simulink model "puma_dy_create_model_ext"  (R2015b)
settings: Solver=FixedStepAuto  StartTime=0.0  StopTime=5  FixedStep=0.01  RelTol=1e-3
values from neighbouring files (symbols this model uses):
  g = 9.80665    [puma_gen_traj_and_mass_param_ext.m]
  ic1 = [ 77887.93599651e-6, -0.00013107e-6, 0.00000935e-6 ... (first row only)    [puma_gen_traj_and_mass_param_ext.m]
  ic2 = [ 214693.97411152e-6, 0, -9732.69714079e-6 ... (first row only)    [puma_gen_traj_and_mass_param_ext.m]
  ic3 = [ 155440.16360976e-6, -7644.06665755e-6, 0.00000000 ... (first row only)    [puma_gen_traj_and_mass_param_ext.m]
  ic4 = [ 2247.32396481e-6, 0.00000000, 0.00000000 ... (first row only)    [puma_gen_traj_and_mass_param_ext.m]
  ic5 = [103.66681738e-6, 0.00000001e-6, -0.00000014e-6 ... (first row only)    [puma_gen_traj_and_mass_param_ext.m]
  ic6 = [311.60326416e-6, -0.00000017e-6, 0.00000000 ... (first row only)    [puma_gen_traj_and_mass_param_ext.m]
  m1 = 12.65615427    [puma_gen_traj_and_mass_param_ext.m]
  m2 = 41.52453758    [puma_gen_traj_and_mass_param_ext.m]
  m3 = 9.95151214    [puma_gen_traj_and_mass_param_ext.m]
  m4 = 1.32832452    [puma_gen_traj_and_mass_param_ext.m]
  m5 = 0.21689844    [puma_gen_traj_and_mass_param_ext.m]
  m6 = 0.32891048    [puma_gen_traj_and_mass_param_ext.m]
  P112 = [ 0 d3 0 ]'    [puma_gen_traj_and_mass_param_ext.m]
  P223 = [ a2 0 0 ]'    [puma_gen_traj_and_mass_param_ext.m]
  P334 = [ a3 d4 0 ]'    [puma_gen_traj_and_mass_param_ext.m]
  P445 = [ 0 0 0 ]'    [puma_gen_traj_and_mass_param_ext.m]
  P556 = [ 0 0 0 ]'    [puma_gen_traj_and_mass_param_ext.m]
  P667 = [ 0 0 0 ]'    [puma_gen_traj_and_mass_param_ext.m]
  Pc111 = [ 0 18.97808196e-3 -4.26387031e-3 ]'    [puma_gen_traj_and_mass_param_ext.m]
  Pc222 = [ 70.91581478e-3 0.00000000 211.69489465e-3-d3 ]'    [puma_gen_traj_and_mass_param_ext.m]
  Pc333 = [ 17.56050216e-3 119.38037782e-3 0 ]'    [puma_gen_traj_and_mass_param_ext.m]
  Pc444 = [ 0 0 -32.52388888e-3 ]'    [puma_gen_traj_and_mass_param_ext.m]
  Pc555 = [ 0 -6.06453643e-3 0 ]'    [puma_gen_traj_and_mass_param_ext.m]
  Pc666 = [ 0 0 93.94499327e-3 ]'    [puma_gen_traj_and_mass_param_ext.m]
libraries: mblibv1 x29
settings Model: Creator=user  LastModifiedBy=qing.hao
settings SimMechanicsCC: VisOnUpdateDiagram=on  VisDuringSimulation=on  LastVizWinPosition=[1 41 1920 938]  CamPosition=[6.48278;4.07346;8.12681;]  CamTarget=[-0.751108;-0.0621973;-0.55549;]  CamUpVector=[-0.477891;-0.569017;0.669208;]  CamHeight=1.40512  VisBackgroundColor=[0.9;0.9;0.95;]  DefaultBodyColor=[1;0;0;]

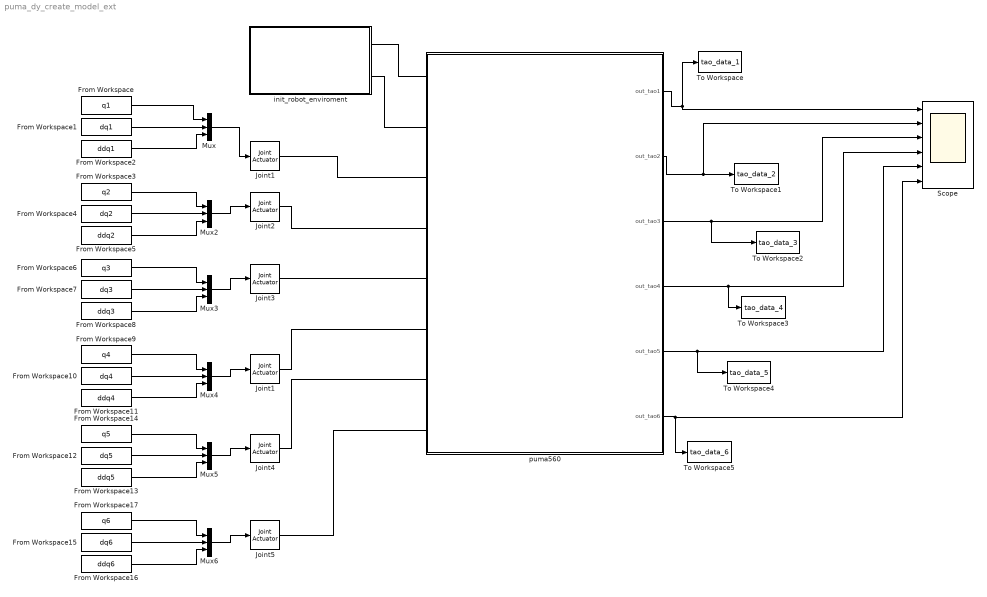
== system puma_dy_create_model_ext ==
  From Workspace : FromWorkspace  VariableName=q1  SampleTime=0.01
  From Workspace1 : FromWorkspace  VariableName=dq1  SampleTime=0.01
  From Workspace10 : FromWorkspace  VariableName=dq4  SampleTime=0.01
  From Workspace11 : FromWorkspace  VariableName=ddq4  SampleTime=0.01
  From Workspace12 : FromWorkspace  VariableName=dq5  SampleTime=0.01
  From Workspace13 : FromWorkspace  VariableName=ddq5  SampleTime=0.01
  From Workspace14 : FromWorkspace  VariableName=q5  SampleTime=0.01
  From Workspace15 : FromWorkspace  VariableName=dq6  SampleTime=0.01
  From Workspace16 : FromWorkspace  VariableName=ddq6  SampleTime=0.01
  From Workspace17 : FromWorkspace  VariableName=q6  SampleTime=0.01
  From Workspace2 : FromWorkspace  VariableName=ddq1  SampleTime=0.01
  From Workspace3 : FromWorkspace  VariableName=q2  SampleTime=0.01
  From Workspace4 : FromWorkspace  VariableName=dq2  SampleTime=0.01
  From Workspace5 : FromWorkspace  VariableName=ddq2  SampleTime=0.01
  From Workspace6 : FromWorkspace  VariableName=q3  SampleTime=0.01
  From Workspace7 : FromWorkspace  VariableName=dq3  SampleTime=0.01
  From Workspace8 : FromWorkspace  VariableName=ddq3  SampleTime=0.01
  From Workspace9 : FromWorkspace  VariableName=q4  SampleTime=0.01
  Joint{1..5} (5 alike) : mblibv1/Sensors &  Actuators/Joint Actuator  UpdateFromCAD=off  PhysicalDomain=Mechanical  PortType=blob  ActuationStyle=Motion  AngleUnits=deg  ArcVelocityUnits=deg/s  ArcAccelerationUnits=deg/s^2  CoordPositionUnits=m  VelocityUnits=m/s  AccelerationUnits=m/s^2  ForceUnits=N  TorqueUnits=N*m  ActiveIO=on  Width=3  DialogClass=MechanicalActuatorBlock  Primitive=R1  ReferenceFrame=Absolute (World)
  "Joint1 " : mblibv1/Sensors &  Actuators/Joint Actuator  UpdateFromCAD=off  PhysicalDomain=Mechanical  PortType=blob  ActuationStyle=Motion  AngleUnits=deg  ArcVelocityUnits=deg/s  ArcAccelerationUnits=deg/s^2  CoordPositionUnits=m  VelocityUnits=m/s  AccelerationUnits=m/s^2  ForceUnits=N  TorqueUnits=N*m  ActiveIO=on  Width=3  DialogClass=MechanicalActuatorBlock  Primitive=R1  ReferenceFrame=Absolute (World)
  Mux{,2..6} (6 alike) : Mux  Inputs=3
  Scope : Scope  NumInputPorts=6
  To Workspace : ToWorkspace  VariableName=tao_data_1  SaveFormat=Timeseries  SampleTime=-1
  To Workspace1 : ToWorkspace  VariableName=tao_data_2  SaveFormat=Timeseries  SampleTime=-1
  To Workspace2 : ToWorkspace  VariableName=tao_data_3  SaveFormat=Timeseries  SampleTime=-1
  To Workspace3 : ToWorkspace  VariableName=tao_data_4  SaveFormat=Timeseries  SampleTime=-1
  To Workspace4 : ToWorkspace  VariableName=tao_data_5  SaveFormat=Timeseries  SampleTime=-1
  To Workspace5 : ToWorkspace  VariableName=tao_data_6  SaveFormat=Timeseries  SampleTime=-1
  "init_robot_enviroment " : Subsystem
  puma560 : Subsystem
  wires:
  From Workspace/1 -> Mux/1
  From Workspace1/1 -> Mux/2
  From Workspace2/1 -> Mux/3
  Mux/1 -> "Joint1 "/1
  From Workspace3/1 -> Mux2/1
  From Workspace4/1 -> Mux2/2
  From Workspace5/1 -> Mux2/3
  Mux2/1 -> Joint2/1
  From Workspace6/1 -> Mux3/1
  From Workspace7/1 -> Mux3/2
  From Workspace8/1 -> Mux3/3
  Mux3/1 -> Joint3/1
  From Workspace9/1 -> Mux4/1
  From Workspace10/1 -> Mux4/2
  From Workspace11/1 -> Mux4/3
  Mux4/1 -> Joint1/1
  From Workspace14/1 -> Mux5/1
  From Workspace12/1 -> Mux5/2
  From Workspace13/1 -> Mux5/3
  Mux5/1 -> Joint4/1
  From Workspace17/1 -> Mux6/1
  From Workspace15/1 -> Mux6/2
  From Workspace16/1 -> Mux6/3
  Mux6/1 -> Joint5/1
  puma560/1(out_tao1) -> To Workspace/1, Scope/1
  puma560/2(out_tao2) -> To Workspace1/1, Scope/2
  puma560/3(out_tao3) -> To Workspace2/1, Scope/3
  puma560/4(out_tao4) -> To Workspace3/1, Scope/4
  puma560/5(out_tao5) -> To Workspace4/1, Scope/5
  puma560/6(out_tao6) -> To Workspace5/1, Scope/6
  connections:
  "Joint1 "/RConn1 -- puma560/LConn3
  puma560/LConn4 -- Joint2/RConn1
  puma560/LConn5 -- Joint3/RConn1
  Joint1/RConn1 -- puma560/LConn6
  Joint4/RConn1 -- puma560/LConn7
  puma560/LConn8 -- Joint5/RConn1
  puma560/LConn1 -- "init_robot_enviroment "/RConn1
  puma560/LConn2 -- "init_robot_enviroment "/RConn2

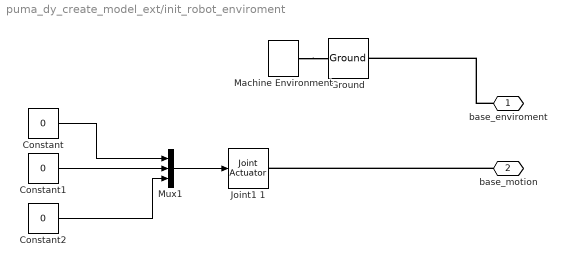
== system puma_dy_create_model_ext/init_robot_enviroment  ==
  Constant : Constant  Value=0
  Constant1 : Constant  Value=0
  Constant2 : Constant  Value=0
  Ground : mblibv1/Bodies/Ground  UpdateFromCAD=off  LeftPortType=env  RightPortType=workingframe  PhysicalDomain=Mechanical  DialogClass=GroundBlock  CoordPosition=[0 0 0]  CoordPositionUnits=m  StateVectorMgrId=3  MachineId=[4 0]  ShowEnvPort=on  ParameterChecksum=[2230059467, 3484987599, 1936103791, 2977691241]  TopologyChecksum=[2683286288, 4268472829, 915100555, 2393938141]
  Joint1 1 : mblibv1/Sensors &  Actuators/Joint Actuator  UpdateFromCAD=off  PhysicalDomain=Mechanical  PortType=blob  ActuationStyle=Motion  AngleUnits=deg  ArcVelocityUnits=deg/s  ArcAccelerationUnits=deg/s^2  CoordPositionUnits=m  VelocityUnits=m/s  AccelerationUnits=m/s^2  ForceUnits=N  TorqueUnits=N*m  ActiveIO=on  Width=3  DialogClass=MechanicalActuatorBlock  Primitive=R1  ReferenceFrame=Absolute (World)
  Machine Environment : mblibv1/Bodies/Machine Environment  PortType=env  PhysicalDomain=Mechanical  DialogTemplateClass=MECH.MachineEnvironment  SyncWhenCopied=off  Gravity=[0 0 -g]  GravityUnits=m/s^2  GravityAsSignal=off  Dimensionality=Auto-detect  AnalysisType=Forward dynamics  LinearAssemblyTolerance=1e-3  LinearAssemblyToleranceUnits=mm  AngularAssemblyTolerance=1e-3  AngularAssemblyToleranceUnits=deg  ConstraintSolverType=Stabilizing  ConstraintRelTolerance=1e-4  ConstraintAbsTolerance=1e-4  UseRobustSingularityHandling=off  RedundancyAnalysisToleranceType=Automatically select tolerance  RedundancyAnalysisTolerance=1e-14  StatePerturbationType=Fixed  PerturbationSize=1e-5  VisualizeMachine=on  BodyVisualizationType=Use model default body geometries  BodyColorSelMode=Use model default  DefaultBodyColor=[1 0 0]
  Mux1 : Mux  Inputs=3
  base_enviroment : PMIOPort  Port=1  Side=Right
  base_motion : PMIOPort  Port=2  Side=Right
  wires:
  Constant1/1 -> Mux1/2
  Constant/1 -> Mux1/1
  Constant2/1 -> Mux1/3
  Mux1/1 -> Joint1 1/1
  connections:
  Machine Environment/RConn1 -- Ground/LConn1
  base_motion/RConn1 -- Joint1 1/RConn1
  base_enviroment/RConn1 -- Ground/RConn1

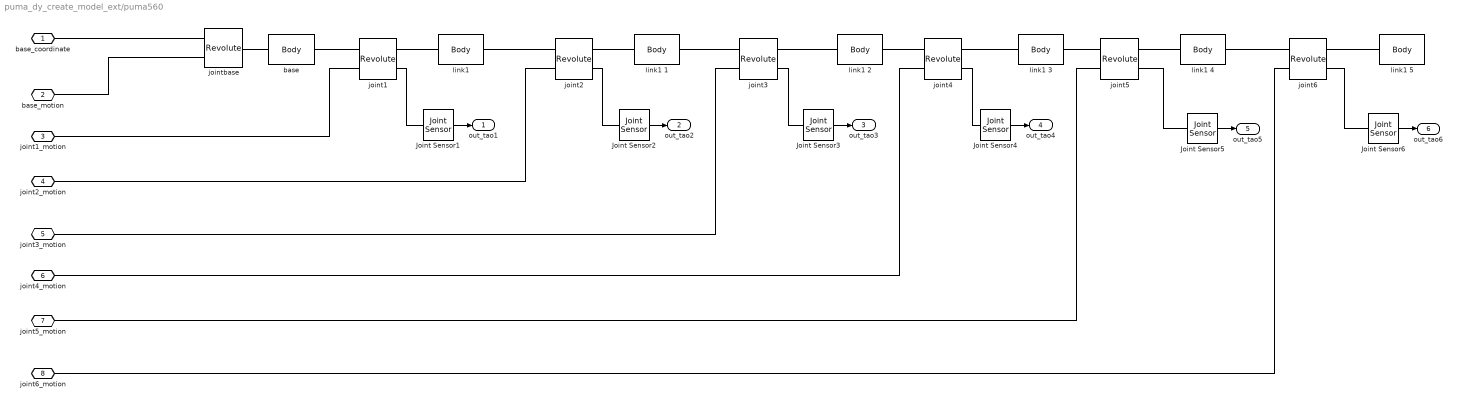
== system puma_dy_create_model_ext/puma560 ==
  Joint Sensor{1..6} (6 alike) : mblibv1/Sensors &  Actuators/Joint Sensor  UpdateFromCAD=off  PhysicalDomain=Mechanical  PortType=blob  Muxed=on  Pose=off  Angle=off  AngleUnits=deg  ArcVelocity=off  ArcVelocityUnits=deg/s  ArcAcceleration=off  ArcAccelerationUnits=deg/s^2  CoordPosition=on  CoordPositionUnits=m  Velocity=off  VelocityUnits=m/s  Acceleration=off  AccelerationUnits=m/s^2  Quaternion=on  QuaternionDT=off  QuaternionDDT=off  QuaternionUnits=off  OutputVector=[1]  ActiveIO=on  Width=1  DialogClass=MechanicalSensorBlock  Primitive=R1  Force=off  ForceUnits=N  Torque=on  TorqueUnits=N*m  ReferenceFrame=Absolute (World)  ReactionSensedSide=Base  ReactionReferenceFrame=Absolute (World)  ReactionForce=off  ReactionForceUnits=N  ReactionMoment=off  ReactionMomentUnits=N*m
  "base " : mblibv1/Bodies/Body  LConnTagsString=CS1  RConnTagsString=CS2  UpdateFromCAD=off  DialogClass=MechanicalBodyBlock  Mass=1  MassUnits=kg  InertiaUnits=kg*m^2  Inertia=eye(3)  Shape=Cylinder  ShapeDims=[1 1]  ShapeUnits=m  ShapeUse=false  Density=1  DensityUnits=kg/m^3  DensityUse=false  GraphicsMode=GFXFILE  GraphicsFileName=.\model\RobotPart0.STL  BodyColorSelMode=COLORPALETTE  BodyColor=[0.87059 0.4902 0]  AttachedToCS=CS3  CG=Left$CG$[0 0 300]$WORLD$WORLD$mm$[0 0 0]$Euler X-Y-Z$deg$WORLD$false$none  WorkingFrames="Left$CS1$[0 0 0]$World$World$mm$[0 0 0]$Euler X-Y-Z$deg$WORLD$true$none#Right$CS2$[0 0  633.57]$World$World$mm$[0 0 0]$Euler X-Y-Z$deg$WORLD$true$none#Right$CS3$[0 -234  0]$World$World$mm$[0 0 0]$Euler X-Y-Z$deg$WORLD$false$none"  CGPos=[0 0 300]  CGRot=[0 0 0]  CS0Pos=[]  CS0Rot=[]  CS1Pos=[0 0 0]  CS1Rot=[0 0 0]  CS2Pos="[0 0  633.57]"  CS2Rot=[0 0 0]  CS3Pos="[0 -234  0]"  CS3Rot=[0 0 0]  CS4Pos=[]  CS4Rot=[]  CS5Pos=[]  CS5Rot=[]  CS6Pos=[]  CS6Rot=[]  CS7Pos=[]  CS7Rot=[]  CS8Pos=[]  CS8Rot=[]  CS9Pos=[]  CS9Rot=[]  CS10Pos=[]  CS10Rot=[]  CS11Pos=[]  CS11Rot=[]  CS12Pos=[]  CS12Rot=[]  CS13Pos=[]  CS13Rot=[]  CS14Pos=[]  CS14Rot=[]  CS15Pos=[]  CS15Rot=[]  CS16Pos=[]  CS16Rot=[]  CS17Pos=[]  CS17Rot=[]  CS18Pos=[]  CS18Rot=[]  CS19Pos=[]  CS19Rot=[]  CS20Pos=[]  CS20Rot=[]
  joint{1..6} (6 alike) : mblibv1/Joints/Revolute  LConnTagsString=__newl0|SA1  RConnTagsString=__newr0|SA1  UpdateFromCAD=off  NumSAPorts=2  CutJoint=off  MarkAsCut=off  Primitives=prismatic  PrimitiveProps=R1$Base$[0 0 1]$revolute  DialogClass=JointBlock  R1Axis=[0 0 1]
  jointbase : mblibv1/Joints/Revolute  LConnTagsString=__newl0|SA1  RConnTagsString=__newr0  UpdateFromCAD=off  NumSAPorts=1  CutJoint=off  MarkAsCut=off  Primitives=prismatic  PrimitiveProps=R1$World$[0 0 1]$revolute  DialogClass=JointBlock  R1Axis=[0 0 1]
  "link1 " : mblibv1/Bodies/Body  LConnTagsString=CS1  RConnTagsString=CS2  UpdateFromCAD=off  DialogClass=MechanicalBodyBlock  Mass=m1  MassUnits=kg  InertiaUnits=kg*m^2  Inertia=ic1  Shape=Cylinder  ShapeDims=[1 1]  ShapeUnits=m  ShapeUse=false  Density=1  DensityUnits=kg/m^3  DensityUse=false  GraphicsMode=GFXFILE  GraphicsFileName=.\model\RobotPart1.STL  BodyColorSelMode=COLORPALETTE  BodyColor=[1 1 0]  AttachedToCS=CS3  CG=Left$CG$Pc111'*1000$CS1$CS1$mm$[0 0 0]$Euler X-Y-Z$deg$CS1$false$none  WorkingFrames=Left$CS1$[0 0 0]$Adjoining$Adjoining$mm$[0 0 0]$Euler X-Y-Z$deg$Adjoining$true$none#Right$CS2$P112'*1000$CS1$CS1$mm$[-90 0 0]$Euler X-Y-Z$deg$CS1$true$none#Right$CS3$[0 -568 0]$World$World$mm$[0 0 0]$Euler X-Y-Z$deg$World$false$none  CGPos=Pc111'*1000  CGRot=[0 0 0]  CS0Pos=[]  CS0Rot=[]  CS1Pos=[0 0 0]  CS1Rot=[0 0 0]  CS2Pos=P112'*1000  CS2Rot=[-90 0 0]  CS3Pos=[0 -568 0]  CS3Rot=[0 0 0]  CS4Pos=[]  CS4Rot=[]  CS5Pos=[]  CS5Rot=[]  CS6Pos=[]  CS6Rot=[]  CS7Pos=[]  CS7Rot=[]  CS8Pos=[]  CS8Rot=[]  CS9Pos=[]  CS9Rot=[]  CS10Pos=[]  CS10Rot=[]  CS11Pos=[]  CS11Rot=[]  CS12Pos=[]  CS12Rot=[]  CS13Pos=[]  CS13Rot=[]  CS14Pos=[]  CS14Rot=[]  CS15Pos=[]  CS15Rot=[]  CS16Pos=[]  CS16Rot=[]  CS17Pos=[]  CS17Rot=[]  CS18Pos=[]  CS18Rot=[]  CS19Pos=[]  CS19Rot=[]  CS20Pos=[]  CS20Rot=[]
  link1 1 : mblibv1/Bodies/Body  LConnTagsString=CS1  RConnTagsString=CS2  UpdateFromCAD=off  DialogClass=MechanicalBodyBlock  Mass=m2  MassUnits=kg  InertiaUnits=kg*m^2  Inertia=ic2  Shape=Cylinder  ShapeDims=[1 1]  ShapeUnits=m  ShapeUse=false  Density=1  DensityUnits=kg/m^3  DensityUse=false  GraphicsMode=GFXFILE  GraphicsFileName=.\model\RobotPart2.STL  BodyColorSelMode=COLORPALETTE  BodyColor=[0.23137 0.44314 0.33726]  AttachedToCS=CS3  CG=Left$CG$Pc222'*1000$CS1$CS1$mm$[0 0 0]$Euler X-Y-Z$deg$CS1$false$none  WorkingFrames=Left$CS1$[0 0 0]$Adjoining$Adjoining$mm$[0 0 0]$Euler X-Y-Z$deg$Adjoining$true$none#Right$CS2$P223'*1000$CS1$CS1$mm$[0 0 0]$Euler X-Y-Z$deg$CS1$true$none#Right$CS3$[0 -568 0]$World$World$mm$[0 0 0]$Euler X-Y-Z$deg$World$false$none  CGPos=Pc222'*1000  CGRot=[0 0 0]  CS0Pos=[]  CS0Rot=[]  CS1Pos=[0 0 0]  CS1Rot=[0 0 0]  CS2Pos=P223'*1000  CS2Rot=[0 0 0]  CS3Pos=[0 -568 0]  CS3Rot=[0 0 0]  CS4Pos=[]  CS4Rot=[]  CS5Pos=[]  CS5Rot=[]  CS6Pos=[]  CS6Rot=[]  CS7Pos=[]  CS7Rot=[]  CS8Pos=[]  CS8Rot=[]  CS9Pos=[]  CS9Rot=[]  CS10Pos=[]  CS10Rot=[]  CS11Pos=[]  CS11Rot=[]  CS12Pos=[]  CS12Rot=[]  CS13Pos=[]  CS13Rot=[]  CS14Pos=[]  CS14Rot=[]  CS15Pos=[]  CS15Rot=[]  CS16Pos=[]  CS16Rot=[]  CS17Pos=[]  CS17Rot=[]  CS18Pos=[]  CS18Rot=[]  CS19Pos=[]  CS19Rot=[]  CS20Pos=[]  CS20Rot=[]
  link1 2 : mblibv1/Bodies/Body  LConnTagsString=CS1  RConnTagsString=CS2  UpdateFromCAD=off  DialogClass=MechanicalBodyBlock  Mass=m3  MassUnits=kg  InertiaUnits=kg*m^2  Inertia=ic3  Shape=Cylinder  ShapeDims=[1 1]  ShapeUnits=m  ShapeUse=false  Density=1  DensityUnits=kg/m^3  DensityUse=false  GraphicsMode=GFXFILE  GraphicsFileName=.\model\RobotPart3.STL  BodyColorSelMode=COLORPALETTE  BodyColor=[1 0 0]  AttachedToCS=CS3  CG=Left$CG$Pc333'*1000$CS1$CS1$mm$[0 0 0]$Euler X-Y-Z$deg$CS1$false$none  WorkingFrames=Left$CS1$[0 0 0]$Adjoining$Adjoining$mm$[0 0 0]$Euler X-Y-Z$deg$Adjoining$true$none#Right$CS2$P334'*1000$CS1$CS1$mm$[-90 0 0]$Euler X-Y-Z$deg$CS1$true$none#Right$CS3$[0 -568 0]$World$World$mm$[0 0 0]$Euler X-Y-Z$deg$World$false$none  CGPos=Pc333'*1000  CGRot=[0 0 0]  CS0Pos=[]  CS0Rot=[]  CS1Pos=[0 0 0]  CS1Rot=[0 0 0]  CS2Pos=P334'*1000  CS2Rot=[-90 0 0]  CS3Pos=[0 -568 0]  CS3Rot=[0 0 0]  CS4Pos=[]  CS4Rot=[]  CS5Pos=[]  CS5Rot=[]  CS6Pos=[]  CS6Rot=[]  CS7Pos=[]  CS7Rot=[]  CS8Pos=[]  CS8Rot=[]  CS9Pos=[]  CS9Rot=[]  CS10Pos=[]  CS10Rot=[]  CS11Pos=[]  CS11Rot=[]  CS12Pos=[]  CS12Rot=[]  CS13Pos=[]  CS13Rot=[]  CS14Pos=[]  CS14Rot=[]  CS15Pos=[]  CS15Rot=[]  CS16Pos=[]  CS16Rot=[]  CS17Pos=[]  CS17Rot=[]  CS18Pos=[]  CS18Rot=[]  CS19Pos=[]  CS19Rot=[]  CS20Pos=[]  CS20Rot=[]
  link1 3 : mblibv1/Bodies/Body  LConnTagsString=CS1  RConnTagsString=CS2  UpdateFromCAD=off  DialogClass=MechanicalBodyBlock  Mass=m4  MassUnits=kg  InertiaUnits=kg*m^2  Inertia=ic4  Shape=Cylinder  ShapeDims=[1 1]  ShapeUnits=m  ShapeUse=false  Density=1  DensityUnits=kg/m^3  DensityUse=false  GraphicsMode=GFXFILE  GraphicsFileName=.\model\RobotPart4.STL  BodyColorSelMode=COLORPALETTE  BodyColor=[0.46667 0.67451 0.18824]  AttachedToCS=CS3  CG=Left$CG$Pc444*1000$CS1$CS1$mm$[0 0 0]$Euler X-Y-Z$deg$CS1$false$none  WorkingFrames=Left$CS1$[0 0 0]$Adjoining$Adjoining$mm$[0 0 0]$Euler X-Y-Z$deg$Adjoining$true$none#Right$CS2$P445'*1000$CS1$CS1$mm$[90 0 0]$Euler X-Y-Z$deg$CS1$true$none#Right$CS3$[0 -568 0]$World$World$mm$[0 0 0]$Euler X-Y-Z$deg$World$false$none  CGPos=Pc444*1000  CGRot=[0 0 0]  CS0Pos=[]  CS0Rot=[]  CS1Pos=[0 0 0]  CS1Rot=[0 0 0]  CS2Pos=P445'*1000  CS2Rot=[90 0 0]  CS3Pos=[0 -568 0]  CS3Rot=[0 0 0]  CS4Pos=[]  CS4Rot=[]  CS5Pos=[]  CS5Rot=[]  CS6Pos=[]  CS6Rot=[]  CS7Pos=[]  CS7Rot=[]  CS8Pos=[]  CS8Rot=[]  CS9Pos=[]  CS9Rot=[]  CS10Pos=[]  CS10Rot=[]  CS11Pos=[]  CS11Rot=[]  CS12Pos=[]  CS12Rot=[]  CS13Pos=[]  CS13Rot=[]  CS14Pos=[]  CS14Rot=[]  CS15Pos=[]  CS15Rot=[]  CS16Pos=[]  CS16Rot=[]  CS17Pos=[]  CS17Rot=[]  CS18Pos=[]  CS18Rot=[]  CS19Pos=[]  CS19Rot=[]  CS20Pos=[]  CS20Rot=[]
  link1 4 : mblibv1/Bodies/Body  LConnTagsString=CS1  RConnTagsString=CS2  UpdateFromCAD=off  DialogClass=MechanicalBodyBlock  Mass=m5  MassUnits=kg  InertiaUnits=kg*m^2  Inertia=ic5  Shape=Cylinder  ShapeDims=[1 1]  ShapeUnits=m  ShapeUse=false  Density=1  DensityUnits=kg/m^3  DensityUse=false  GraphicsMode=GFXFILE  GraphicsFileName=.\model\RobotPart5.STL  BodyColorSelMode=COLORPALETTE  BodyColor=[0 0 0]  AttachedToCS=CS3  CG=Left$CG$Pc555*1000$CS1$CS1$mm$[0 0 0]$Euler X-Y-Z$deg$CS1$false$none  WorkingFrames=Left$CS1$[0 0 0]$Adjoining$Adjoining$mm$[0 0 0]$Euler X-Y-Z$deg$Adjoining$true$none#Right$CS2$P556'*1000$CS1$CS1$mm$[-90 0 0]$Euler X-Y-Z$deg$CS1$true$none#Right$CS3$[0 -568 0]$World$World$mm$[0 0 0]$Euler X-Y-Z$deg$World$false$none  CGPos=Pc555*1000  CGRot=[0 0 0]  CS0Pos=[]  CS0Rot=[]  CS1Pos=[0 0 0]  CS1Rot=[0 0 0]  CS2Pos=P556'*1000  CS2Rot=[-90 0 0]  CS3Pos=[0 -568 0]  CS3Rot=[0 0 0]  CS4Pos=[]  CS4Rot=[]  CS5Pos=[]  CS5Rot=[]  CS6Pos=[]  CS6Rot=[]  CS7Pos=[]  CS7Rot=[]  CS8Pos=[]  CS8Rot=[]  CS9Pos=[]  CS9Rot=[]  CS10Pos=[]  CS10Rot=[]  CS11Pos=[]  CS11Rot=[]  CS12Pos=[]  CS12Rot=[]  CS13Pos=[]  CS13Rot=[]  CS14Pos=[]  CS14Rot=[]  CS15Pos=[]  CS15Rot=[]  CS16Pos=[]  CS16Rot=[]  CS17Pos=[]  CS17Rot=[]  CS18Pos=[]  CS18Rot=[]  CS19Pos=[]  CS19Rot=[]  CS20Pos=[]  CS20Rot=[]
  link1 5 : mblibv1/Bodies/Body  LConnTagsString=CS1  RConnTagsString=CS2  UpdateFromCAD=off  DialogClass=MechanicalBodyBlock  Mass=m6  MassUnits=kg  InertiaUnits=kg*m^2  Inertia=ic6  Shape=Cylinder  ShapeDims=[1 1]  ShapeUnits=m  ShapeUse=false  Density=1  DensityUnits=kg/m^3  DensityUse=false  GraphicsMode=GFXFILE  GraphicsFileName=.\model\RobotPart6.STL  BodyColorSelMode=COLORPALETTE  BodyColor=[0 0 1]  AttachedToCS=CS3  CG=Left$CG$Pc666*1000$CS1$CS1$mm$[0 0 0]$Euler X-Y-Z$deg$CS1$false$none  WorkingFrames=Left$CS1$[0 0 0]$Adjoining$Adjoining$mm$[0 0 0]$Euler X-Y-Z$deg$Adjoining$true$none#Right$CS2$P667'*1000$CS1$CS1$mm$[0 0 0]$Euler X-Y-Z$deg$CS1$true$none#Right$CS3$[0 -568 0]$World$World$mm$[0 0 0]$Euler X-Y-Z$deg$World$false$none  CGPos=Pc666*1000  CGRot=[0 0 0]  CS0Pos=[]  CS0Rot=[]  CS1Pos=[0 0 0]  CS1Rot=[0 0 0]  CS2Pos=P667'*1000  CS2Rot=[0 0 0]  CS3Pos=[0 -568 0]  CS3Rot=[0 0 0]  CS4Pos=[]  CS4Rot=[]  CS5Pos=[]  CS5Rot=[]  CS6Pos=[]  CS6Rot=[]  CS7Pos=[]  CS7Rot=[]  CS8Pos=[]  CS8Rot=[]  CS9Pos=[]  CS9Rot=[]  CS10Pos=[]  CS10Rot=[]  CS11Pos=[]  CS11Rot=[]  CS12Pos=[]  CS12Rot=[]  CS13Pos=[]  CS13Rot=[]  CS14Pos=[]  CS14Rot=[]  CS15Pos=[]  CS15Rot=[]  CS16Pos=[]  CS16Rot=[]  CS17Pos=[]  CS17Rot=[]  CS18Pos=[]  CS18Rot=[]  CS19Pos=[]  CS19Rot=[]  CS20Pos=[]  CS20Rot=[]
  base_coordinate : PMIOPort  Port=1  Side=Left
  base_motion : PMIOPort  Port=2  Side=Left
  "joint1_motion " : PMIOPort  Port=3  Side=Left
  joint2_motion : PMIOPort  Port=4  Side=Left
  joint3_motion : PMIOPort  Port=5  Side=Left
  joint4_motion : PMIOPort  Port=6  Side=Left
  joint5_motion : PMIOPort  Port=7  Side=Left
  joint6_motion : PMIOPort  Port=8  Side=Left
  out_tao1 : Outport
  out_tao2 : Outport  Port=2
  out_tao3 : Outport  Port=3
  out_tao4 : Outport  Port=4
  out_tao5 : Outport  Port=5
  out_tao6 : Outport  Port=6
  wires:
  Joint Sensor1/1 -> out_tao1/1
  Joint Sensor2/1 -> out_tao2/1
  Joint Sensor3/1 -> out_tao3/1
  Joint Sensor4/1 -> out_tao4/1
  Joint Sensor5/1 -> out_tao5/1
  Joint Sensor6/1 -> out_tao6/1
  connections:
  jointbase/RConn1 -- "base "/LConn1
  jointbase/LConn1 -- base_coordinate/RConn1
  jointbase/LConn2 -- base_motion/RConn1
  "base "/RConn1 -- joint1/LConn1
  "joint1_motion "/RConn1 -- joint1/LConn2
  Joint Sensor1/LConn1 -- joint1/RConn2
  joint1/RConn1 -- "link1 "/LConn1
  joint2/RConn1 -- link1 1/LConn1
  Joint Sensor2/LConn1 -- joint2/RConn2
  joint2/LConn1 -- "link1 "/RConn1
  joint2/LConn2 -- joint2_motion/RConn1
  joint3/LConn1 -- link1 1/RConn1
  joint3/LConn2 -- joint3_motion/RConn1
  link1 2/LConn1 -- joint3/RConn1
  joint3/RConn2 -- Joint Sensor3/LConn1
  joint4/LConn1 -- link1 2/RConn1
  link1 3/LConn1 -- joint4/RConn1
  joint4/LConn2 -- joint4_motion/RConn1
  joint4/RConn2 -- Joint Sensor4/LConn1
  joint5/LConn1 -- link1 3/RConn1
  joint5/LConn2 -- joint5_motion/RConn1
  link1 4/LConn1 -- joint5/RConn1
  joint5/RConn2 -- Joint Sensor5/LConn1
  joint6/LConn1 -- link1 4/RConn1
  joint6/LConn2 -- joint6_motion/RConn1
  joint6/RConn2 -- Joint Sensor6/LConn1
  link1 5/LConn1 -- joint6/RConn1
